simulink model "LoggingModel"  (R2017a)
settings: Solver=FixedStepAuto  StartTime=0.0  StopTime=10.0  RelTol=1e-3
values from neighbouring files (symbols this model uses):
  EnableLogging = Simulink.Parameter    [CreateParameter.m]
undefined symbols (not defined in the file or in its folder): DiscIntNeverNeededParam
settings Model: Creator=darenlee  LastModifiedBy=darenlee
settings SolverCC: PositivePriorityOrder=on
settings OptimizationCC: MaxStackSize=64
settings DebuggingCC: ParameterTunabilityLossMsg=error
settings SFSimCC: MATLABDynamicMemAlloc=off
settings RTWCC: SystemTargetFile=ert.tlc  HardwareBoard=QNX-x86  TLCOptions="-aInlineSetEventsForThisBaseRateFcn=TLC_FALSE -aSuppressMultiTaskScheduler=TLC_FALSE  -aRateBasedStepFcn=0"  TemplateMakefile=ert_default_tmf  Description=Embedded Coder  GenerateReport=on  Toolchain=QNX QCC Toolchain  IncludeHyperlinkInReport=on  LaunchReport=on  GenerateTraceInfo=on  GenerateTraceReport=on  GenerateTraceReportSl=on  GenerateTraceReportSf=on  GenerateTraceReportEml=on
settings CodeAppCC: ForceParamTrailComments=on  IgnoreCustomStorageClasses=off  OperatorAnnotations=on  SimulinkDataObjDesc=on  SFDataObjDesc=on  MATLABFcnDesc=on  InsertBlockDesc=on  MATLABSourceComments=on
settings ERTTargetCC: MultiwordLength=2048

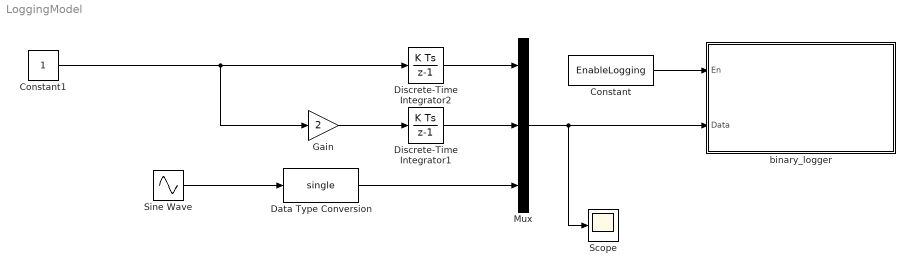
== system LoggingModel ==
  Constant : Constant  Value=EnableLogging  OutDataTypeStr=boolean  SampleTime=-1
  Constant1 : Constant  OutDataTypeStr=single
  Data Type Conversion : DataTypeConversion  OutDataTypeStr=single
  Discrete-Time Integrator1 : DiscreteIntegrator  InitialConditionSetting=State (most efficient)  SampleTime=-1  ICPrevOutput=DiscIntNeverNeededParam  ICPrevScaledInput=DiscIntNeverNeededParam
  Discrete-Time Integrator2 : DiscreteIntegrator  InitialConditionSetting=State (most efficient)  SampleTime=-1  ICPrevOutput=DiscIntNeverNeededParam  ICPrevScaledInput=DiscIntNeverNeededParam
  Gain : Gain  Gain=2  OutDataTypeStr=Inherit: Same as input
  Mux : Mux  Inputs=3
  Scope : Scope
  Sine Wave : Sin  SampleTime=0.1
  binary_logger : Subsystem  mask(Pixhawk Binary Logger){logfile=/tmp/bin_log, cacheflag=on, numRecs=10}
      mask prompts: cacheflag "Cache in Memory"; numRecs "Max Record Count"
      mask help:
      | Log a vector of data to a file on the SD card
      | If Cache in Memory is on data is written when en goes low or when max number of records specified is reached.
      | Otherwise Max Number of Records is used to indicate when to performa an fflush out to file.
      mask init:
      | logname=uint8(logfile);
      mask Display:
      | fprintf(get_param(gcb,'logfile'))
      | port_label('input',1,'en')
      | port_label('input',2,'data')
  wires:
  Discrete-Time Integrator1/1 -> Mux/2
  Gain/1 -> Discrete-Time Integrator1/1
  Constant1/1 -> Gain/1, Discrete-Time Integrator2/1
  Discrete-Time Integrator2/1 -> Mux/1
  Constant/1 -> binary_logger/1(En)
  Mux/1 -> Scope/1, binary_logger/2(Data)
  Sine Wave/1 -> Data Type Conversion/1
  Data Type Conversion/1 -> Mux/3

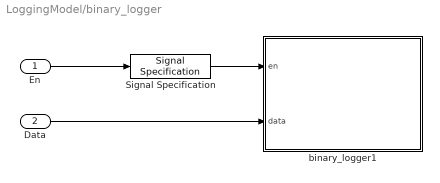
== system LoggingModel/binary_logger ==
  En : Inport
  Data : Inport  Port=2
  Signal Specification : SignalSpecification  OutDataTypeStr=boolean
  binary_logger1 : MATLAB Function  TreatAsAtomicUnit=on
  wires:
  Data/1 -> binary_logger1/2(data)
  En/1 -> Signal Specification/1
  Signal Specification/1 -> binary_logger1/1(en)

== matlab function LoggingModel/binary_logger/binary_logger1 ==
  data: en input boolean; data input; logname parameter uint8; cacheflag parameter boolean; numRecs parameter uint32
%% Binary Logger
% Note: All data needs to be of the same type (e.g. double)
% Header information format:
%           String "MWLOGV##"
%           Time/Date 4 bytes (time())
%           Number of Signals per record Logged 1 byte (256 max)
%           Data Type of Signals Logged  1 byte (1-10)
%           Number of bytes per record 2 bytes (65535 max)
% This does NOT include the number of data sets logged.  
% i.e. The Reader is responsible for reading until EOF.
% MathWorks Pilot Engineering 2015
% Steve Kuznicki
function binary_logger(en, data, logname, cacheflag, numRecs)
%#codegen
    persistent fp isflushed isopen count lognumstr elem_size vect_size datastore
    coder.cinclude('<stdio.h>');
    coder.cinclude('<time.h>');

    if isempty(count)
        count = uint32(0);
        lognumstr = 65;
        isopen = false;
        fp = coder.opaque('FILE*', 'NULL');
        isflushed = false;
        elem_size = uint16(1);
        vect_size = coder.const(uint8(numel(data)));
        if cacheflag == true
            datastore = zeros(numRecs*uint32(coder.const(numel(data))), 1, 'like', data);
        end
    end

    if (en)
        if isopen == false
            [elsize, eltype] = get_elem_size(data);
            elem_size = coder.const(uint16(elsize));
            elem_type = coder.const(uint8(eltype));
            vect_size = coder.const(uint8(numel(data)));
            coder.ceval('printf',['OPENING file %s vect_size %d elem_size %d numRecs %d %c' uint8(0)], ...
                [logname, '_', char(lognumstr), '.bin', int8(0)], uint32(vect_size), uint32(elem_size), uint32(numRecs), uint8(10));
            fp = coder.ceval('fopen', [logname, '_', char(lognumstr), '.bin', int8(0)], ['wb', int8(0)]);
            lognumstr = lognumstr + 1;
            isflushed = false;
            count = uint32(0);
            isopen = true;
            % Write header information here
            % header token + version
            mlStrVer = 'MWLOGV01';
            coder.ceval('fwrite', coder.rref(mlStrVer), uint32(1), length(mlStrVer), fp);
            % date/time
            tm = uint32(0);
            tmptr = uint32(0);
            tm = coder.ceval('time',coder.wref(tmptr));
            coder.ceval('fwrite', coder.rref(tm), uint32(4), uint32(1), fp);
            % number of elements in each record
            coder.ceval('fwrite', coder.rref(vect_size), uint32(1), uint32(1), fp);
            % data type of the elements
            coder.ceval('fwrite', coder.rref(elem_type), uint32(1), uint32(1), fp);
            % size of each record in bytes
            recSize = elem_size * uint16(vect_size);
            coder.ceval('fwrite', coder.rref(recSize), uint32(2), uint32(1), fp);
        end
        % cache data in memory or use fwrite
        if cacheflag == true
            addr = (count*uint32(vect_size))+1;
            for idx = 1:vect_size
                datastore(addr) = data(idx);
                addr = addr + 1;
            end
        else
            coder.ceval('fwrite', coder.rref(data), elem_size, vect_size, fp);
        end
        count = count + uint32(1);
        % check for data count limit
        if count >= numRecs
            if cacheflag
                for idx = 1:count*uint32(vect_size)
                    coder.ceval('fwrite', coder.rref(datastore(idx)), elem_size, uint32(1), fp);
                end
            end
            coder.ceval('fflush', fp);
            isflushed = false;
            count = uint32(0);
        end
    else
        if isopen == true
            if ~isflushed
                coder.ceval('printf',['CLOSING file. count = %d %c' uint8(0)], uint32(count), uint8(10));
                if cacheflag
                    count = count + uint32(1);
                    for idx = 1:count*uint32(vect_size)
                        coder.ceval('fwrite', coder.rref(datastore(idx)), elem_size, uint32(1), fp);
                    end
                end
                coder.ceval('fflush', fp);
                isflushed = true;
            end
            coder.ceval('fclose', fp);
        end
        isopen = false;
        count = uint32(0);
    end
end

% return the size of the element in bytes
function [elem_size, dtype] = get_elem_size(data)
    switch(class(data))
        case 'double'
            elem_size = 8;
            dtype = 1;
        case 'single'
            elem_size = 4;
            dtype = 2;
        case 'int32'
            elem_size = 4;
            dtype = 3;
        case 'uint32'
            elem_size = 4;
            dtype = 4;
        case 'int16'
            elem_size = 2;
            dtype = 5;
        case 'uint16'
            elem_size = 2;
            dtype = 6;
        case 'int8'
            elem_size = 1;
            dtype = 7;
        case 'uint8'
            elem_size = 1;
            dtype = 8;
        case 'logical'
            elem_size = 1;
            dtype = 9;
        case 'embedded.fi'
            nt = numerictype(data);
            elem_size = 2^ceil(log2(ceil(nt.WordLength / 8)));
            dtype = 10;
    end
    if ~isreal(data)
        elem_size = elem_size*2;
    end
    
    elem_size = uint16(elem_size);
    dtype = uint8(dtype);
end
